simulink model "bdotController_test"  (R2018b)
settings: Solver=VariableStepAuto  StartTime=0.0  StopTime=5400  MaxStep=0.005  RelTol=1e-3
undefined symbols (not defined in the file): simParams
libraries: aerolibutil x3, vrlib x2, mtq_lib x2, sharedutil x1, battery_lib x1, bdotController_lib x1, teme2eci_lib x1, clock_lib x1, time_Lib x1, magField_lib x1, sgp4_lib_fsw x1, solar_panels_lib x1
settings Model: Creator=taylorreynolds  LastModifiedBy=Taylor

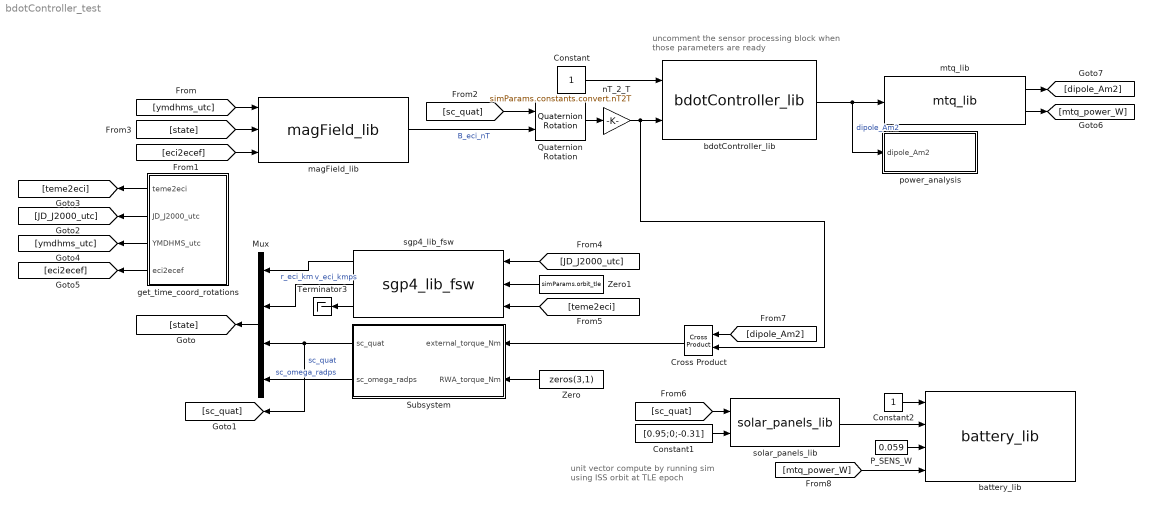
== system bdotController_test ==
  note: unit vector compute by running sim
      | using ISS orbit at TLE epoch
  note: uncomment the sensor processing block
      | when those parameters are ready
  Constant : Constant
  Constant1 : Constant  Value=[0.95;0;-0.31]
  Constant2 : Constant
  Cross Product : vrlib/Utilities/Cross Product
      settings: SourceProductBaseCode=VR
  Mux : Mux  Inputs=[3 3 4 3]
  "P_SENS_W " : Constant  Value=0.059
  Quaternion Rotation : aerolibutil/Quaternion Rotation
  Subsystem : Subsystem
  Terminator3 : Terminator
  Zero : Constant  Value=zeros(3,1)  OutDataTypeStr=Inherit: Inherit via back propagation
  Zero1 : Constant  Value=simParams.orbit_tle  OutDataTypeStr=Inherit: Inherit via back propagation
  battery_lib : battery_lib/battery_lib  SystemSampleTime=-1
  bdotController_lib : bdotController_lib/bdotController_lib  SystemSampleTime=-1
  get_time_coord_rotations : Subsystem
  magField_lib : magField_lib/magField_lib  SystemSampleTime=-1
  mtq_lib : mtq_lib/mtq_lib  SystemSampleTime=-1
  nT_2_T : Gain  Gain=simParams.constants.convert.nT2T
  "power_analysis " : Subsystem
  sgp4_lib_fsw : sgp4_lib_fsw/sgp4_lib_fsw  SystemSampleTime=-1
  solar_panels_lib : solar_panels_lib/solar_panels_lib  SystemSampleTime=-1
  wires:
  Constant/1 -> bdotController_lib/1
  bdotController_lib/1 -> "power_analysis "/1(dipole_Am2), mtq_lib/1  "dipole_Am2"
  Cross Product/1 -> Subsystem/1(external_torque_Nm)
  Mux/1 -> [state]
  Zero/1 -> Subsystem/2(RWA_torque_Nm)
  [state] -> magField_lib/2
  nT_2_T/1 -> bdotController_lib/2, Cross Product/2
  [ymdhms_utc] -> magField_lib/1
  [eci2ecef] -> magField_lib/3
  Subsystem/1(sc_quat) -> [sc_quat], Mux/3  "sc_quat"
  Subsystem/2(sc_omega_radps) -> Mux/4  "sc_omega_radps"
  sgp4_lib_fsw/1 -> Mux/1  "r_eci_km"
  sgp4_lib_fsw/2 -> Mux/2  "v_eci_kmps"
  magField_lib/1 -> Quaternion Rotation/2  "B_eci_nT"
  [sc_quat] -> Quaternion Rotation/1
  Quaternion Rotation/1 -> nT_2_T/1
  sgp4_lib_fsw/3 -> Terminator3/1
  Zero1/1 -> sgp4_lib_fsw/2
  [JD_J2000_utc] -> sgp4_lib_fsw/1
  get_time_coord_rotations/3(YMDHMS_utc) -> [ymdhms_utc]
  get_time_coord_rotations/2(JD_J2000_utc) -> [JD_J2000_utc]
  get_time_coord_rotations/1(teme2eci) -> [teme2eci]
  [teme2eci] -> sgp4_lib_fsw/3
  get_time_coord_rotations/4("eci2ecef ") -> [eci2ecef]
  [sc_quat] -> solar_panels_lib/1
  Constant1/1 -> solar_panels_lib/2
  solar_panels_lib/1 -> battery_lib/2
  Constant2/1 -> battery_lib/1
  "P_SENS_W "/1 -> battery_lib/3
  mtq_lib/2 -> [mtq_power_W]
  mtq_lib/1 -> [dipole_Am2]
  [dipole_Am2] -> Cross Product/1
  [mtq_power_W] -> battery_lib/4

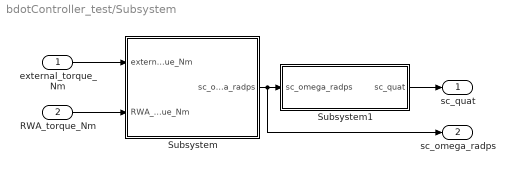
== system bdotController_test/Subsystem ==
  external_torque_Nm : Inport
  RWA_torque_Nm : Inport  Port=2
  Subsystem : Subsystem
  Subsystem1 : Subsystem
  sc_quat : Outport
  sc_omega_radps : Outport  Port=2
  wires:
  external_torque_Nm/1 -> Subsystem/1(external_torque_Nm)
  RWA_torque_Nm/1 -> Subsystem/2(RWA_torque_Nm)
  Subsystem/1(sc_omega_radps) -> sc_omega_radps/1, Subsystem1/1(sc_omega_radps)
  Subsystem1/1(sc_quat) -> sc_quat/1

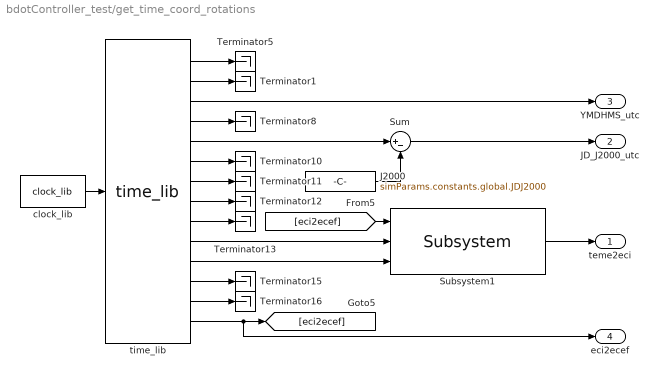
== system bdotController_test/get_time_coord_rotations ==
  J2000 : Constant  Value=simParams.constants.global.JDJ2000  OutDataTypeStr=Inherit: Inherit via back propagation
  Subsystem1 : teme2eci_lib/Subsystem  SystemSampleTime=-1
  Sum : Sum  Inputs=|+-
  Terminator{1,5,8,10..13,15..16} (9 alike) : Terminator
  clock_lib : clock_lib/clock_lib  SystemSampleTime=-1
  "time_lib " : time_Lib/time_lib    SystemSampleTime=-1
  teme2eci : Outport
  JD_J2000_utc : Outport  Port=2
  YMDHMS_utc : Outport  Port=3
  "eci2ecef " : Outport  Port=4
  wires:
  "time_lib "/11 -> Subsystem1/3
  [eci2ecef] -> Subsystem1/1
  J2000/1 -> Sum/2
  "time_lib "/10 -> Subsystem1/2
  "time_lib "/6 -> Terminator10/1
  "time_lib "/13 -> Terminator16/1
  clock_lib/1 -> "time_lib "/1
  "time_lib "/3 -> YMDHMS_utc/1
  "time_lib "/7 -> Terminator11/1
  "time_lib "/2 -> Terminator1/1
  "time_lib "/5 -> Sum/1
  "time_lib "/14 -> "eci2ecef "/1, [eci2ecef]
  "time_lib "/12 -> Terminator15/1
  "time_lib "/1 -> Terminator5/1
  "time_lib "/4 -> Terminator8/1
  "time_lib "/8 -> Terminator12/1
  "time_lib "/9 -> Terminator13/1
  Subsystem1/1 -> teme2eci/1
  Sum/1 -> JD_J2000_utc/1

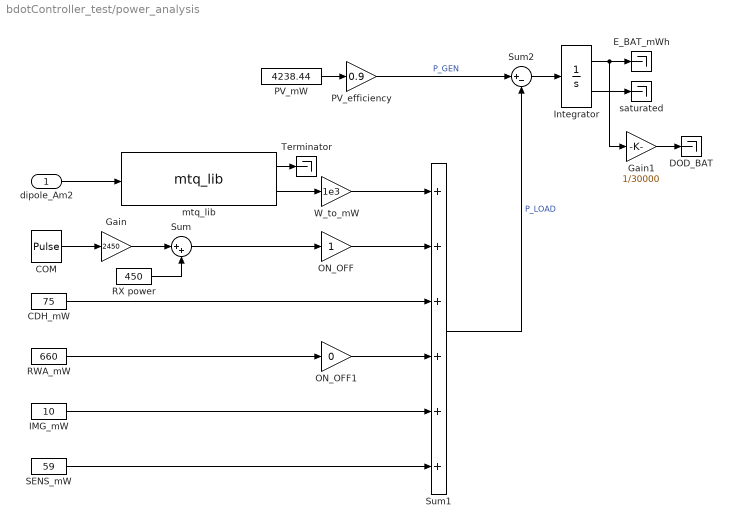
== system bdotController_test/power_analysis  ==
  dipole_Am2 : Inport
  "CDH_mW " : Constant  Value=75
  "COM " : DiscretePulseGenerator  PulseType=Time based  Period=60  PulseWidth=5
  DOD_BAT : Terminator
  E_BAT_mWh : Terminator
  Gain : Gain  Gain=2450
  Gain1 : Gain  Gain=1/30000
  IMG_mW : Constant  Value=10
  Integrator : Integrator  InitialCondition=30000  LimitOutput=on  UpperSaturationLimit=30000  LowerSaturationLimit=0  ShowSaturationPort=on
  ON_OFF : Gain
  ON_OFF1 : Gain  Gain=0
  PV_efficiency : Gain  Gain=0.9
  "PV_mW " : Constant  Value=4238.44
  RWA_mW : Constant  Value=660
  RX power : Constant  Value=450
  "SENS_mW " : Constant  Value=59
  Sum : Sum  Inputs=|++
  Sum1 : Sum  Inputs=++++++
  Sum2 : Sum  Inputs=|+-
  Terminator : Terminator
  W_to_mW : Gain  Gain=1e3
  mtq_lib : mtq_lib/mtq_lib  SystemSampleTime=-1
  saturated : Terminator
  wires:
  dipole_Am2/1 -> mtq_lib/1
  mtq_lib/2 -> W_to_mW/1
  "COM "/1 -> Gain/1
  Gain/1 -> Sum/1
  RX power/1 -> Sum/2
  Sum/1 -> ON_OFF/1
  W_to_mW/1 -> Sum1/1
  mtq_lib/1 -> Terminator/1
  "PV_mW "/1 -> PV_efficiency/1
  PV_efficiency/1 -> Sum2/1  "P_GEN"
  "CDH_mW "/1 -> Sum1/3
  RWA_mW/1 -> ON_OFF1/1
  IMG_mW/1 -> Sum1/5
  "SENS_mW "/1 -> Sum1/6
  Sum1/1 -> Sum2/2  "P_LOAD"
  Sum2/1 -> Integrator/1
  Integrator/1 -> Gain1/1, E_BAT_mWh/1
  Integrator/2 -> saturated/1
  ON_OFF/1 -> Sum1/2
  ON_OFF1/1 -> Sum1/4
  Gain1/1 -> DOD_BAT/1

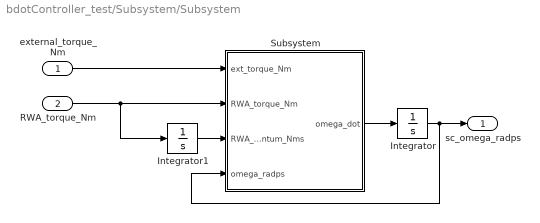
== system bdotController_test/Subsystem/Subsystem ==
  external_torque_Nm : Inport
  RWA_torque_Nm : Inport  Port=2
  Integrator : Integrator  InitialCondition=simParams.initialConditions.w0
  Integrator1 : Integrator
  Subsystem : Subsystem
  sc_omega_radps : Outport
  wires:
  RWA_torque_Nm/1 -> Integrator1/1, Subsystem/2(RWA_torque_Nm)
  external_torque_Nm/1 -> Subsystem/1(ext_torque_Nm)
  Integrator1/1 -> Subsystem/3(RWA_momentum_Nms)
  Subsystem/1(omega_dot) -> Integrator/1
  Integrator/1 -> Subsystem/4(omega_radps), sc_omega_radps/1

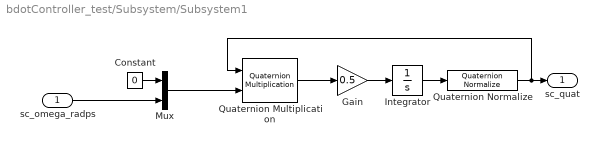
== system bdotController_test/Subsystem/Subsystem1 ==
  sc_omega_radps : Inport
  Constant : Constant  Value=0
  Gain : Gain  Gain=0.5
  Integrator : Integrator  InitialCondition=simParams.initialConditions.q0
  Mux : Mux  Inputs=[1 3]
  Quaternion Multiplication : aerolibutil/Quaternion Multiplication
  Quaternion Normalize : sharedutil/Quaternion Normalize  aMode=aMode
      settings: SourceProductName=Aerospace Blockset  SourceProductBaseCode=AE
  sc_quat : Outport
  wires:
  sc_omega_radps/1 -> Mux/2
  Constant/1 -> Mux/1
  Mux/1 -> Quaternion Multiplication/2
  Quaternion Multiplication/1 -> Gain/1
  Gain/1 -> Integrator/1
  Integrator/1 -> Quaternion Normalize/1
  Quaternion Normalize/1 -> Quaternion Multiplication/1, sc_quat/1

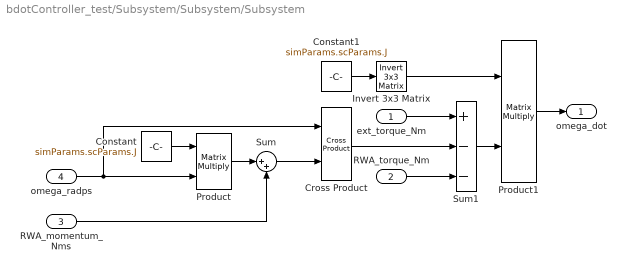
== system bdotController_test/Subsystem/Subsystem/Subsystem ==
  ext_torque_Nm : Inport
  RWA_torque_Nm : Inport  Port=2
  RWA_momentum_Nms : Inport  Port=3
  omega_radps : Inport  Port=4
  Constant : Constant  Value=simParams.scParams.J
  Constant1 : Constant  Value=simParams.scParams.J
  Cross Product : vrlib/Utilities/Cross Product
      settings: SourceProductBaseCode=VR
  Invert 3x3 Matrix : aerolibutil/Invert  3x3 Matrix
  Product : Product  Multiplication=Matrix(*)
  Product1 : Product  Multiplication=Matrix(*)
  Sum : Sum  Inputs=|++
  Sum1 : Sum  Inputs=+--
  omega_dot : Outport
  wires:
  Constant/1 -> Product/1
  omega_radps/1 -> Cross Product/1, Product/2
  Product/1 -> Sum/1
  RWA_momentum_Nms/1 -> Sum/2
  Sum/1 -> Cross Product/2
  Cross Product/1 -> Sum1/2
  RWA_torque_Nm/1 -> Sum1/3
  ext_torque_Nm/1 -> Sum1/1
  Constant1/1 -> Invert 3x3 Matrix/1
  Invert 3x3 Matrix/1 -> Product1/1
  Sum1/1 -> Product1/2
  Product1/1 -> omega_dot/1
